simulink model "CoETM_ClgDem"  (R2016b)
settings: configuration reference "CodeGenConfigSet" (kept outside this file)
values from neighbouring files (symbols this model uses):
  CoETM_AfterRun2_C = Calibration.Parameter    [init_CoETM_ClgDem.m]
  CoETM_facAftRun2_C = Calibration.Parameter    [init_CoETM_ClgDem.m]
  CoETM_facClgAftRun_CUR = Calibration.Parameter    [init_CoETM_ClgDem.m]
  CoETM_facClgAftRun_CURX = Calibration.Parameter    [init_CoETM_ClgDem.m]
  CoETM_facClgDem_DT_C = Calibration.Parameter    [init_CoETM_ClgDem.m]
  CoETM_rClgAftRun_MAP = Calibration.Parameter    [init_CoETM_ClgDem.m]
  CoETM_rClgAftRun_MAPX = Calibration.Parameter    [init_CoETM_ClgDem.m]
  CoETM_rClgAftRun_MAPY = Calibration.Parameter    [init_CoETM_ClgDem.m]
  CoETM_rClgDemFan_CUR = Calibration.Parameter    [init_CoETM_ClgDem.m]
  CoETM_rClgDemFan_CURX = Calibration.Parameter    [init_CoETM_ClgDem.m]
  CoETM_rClgDemMax_C = Calibration.Parameter    [init_CoETM_ClgDem.m]
  CoETM_rClgDemMin_C = Calibration.Parameter    [init_CoETM_ClgDem.m]
  CoETM_rClgDemT_CUR = Calibration.Parameter    [init_CoETM_ClgDem.m]
  CoETM_rClgDemT_CURX = Calibration.Parameter    [init_CoETM_ClgDem.m]
  CoETM_rClgKi_CUR = Calibration.Parameter    [init_CoETM_ClgDem.m]
  CoETM_rClgKi_CURX = Calibration.Parameter    [init_CoETM_ClgDem.m]
  CoETM_rClgKp_CUR = Calibration.Parameter    [init_CoETM_ClgDem.m]
  CoETM_rClgKp_CURX = Calibration.Parameter    [init_CoETM_ClgDem.m]
  CoETM_RmpSlpNeg_C = Calibration.Parameter    [init_CoETM_ClgDem.m]
  CoETM_RmpSlpPos_C = Calibration.Parameter    [init_CoETM_ClgDem.m]
  CoETM_swtCTTCTL_SY_C = Calibration.Parameter    [init_CoETM_ClgDem.m]
  CoETM_swtSrc_C = Calibration.Parameter    [init_CoETM_ClgDem.m]
  CoETM_tAftRunAbrt_C = Calibration.Parameter    [init_CoETM_ClgDem.m]
  CoETM_tClntStg1Max_C = Calibration.Parameter    [init_CoETM_ClgDem.m]
  CoETM_tClntStg1Min_C = Calibration.Parameter    [init_CoETM_ClgDem.m]
  CoETM_tClntStg2Max_C = Calibration.Parameter    [init_CoETM_ClgDem.m]
  CoETM_tClntStg2Min_C = Calibration.Parameter    [init_CoETM_ClgDem.m]
  CoETM_tDvtMax_C = Calibration.Parameter    [init_CoETM_ClgDem.m]
  CoETM_tDvtMin_C = Calibration.Parameter    [init_CoETM_ClgDem.m]
  CoETM_tDvtStg0_C = Calibration.Parameter    [init_CoETM_ClgDem.m]
  CoETM_tDvtStg1_C = Calibration.Parameter    [init_CoETM_ClgDem.m]
  CoETM_tDvtStg2_C = Calibration.Parameter    [init_CoETM_ClgDem.m]
  CoETM_tEngOutSubsOff_C = Calibration.Parameter    [init_CoETM_ClgDem.m]
  CoETM_tiClgAftRun2_MAP = Calibration.Parameter    [init_CoETM_ClgDem.m]
  CoETM_tiClgAftRun2_MAPX = Calibration.Parameter    [init_CoETM_ClgDem.m]
  CoETM_tiClgAftRun2_MAPY = Calibration.Parameter    [init_CoETM_ClgDem.m]
  CoETM_tiClgAftRun_MAP = Calibration.Parameter    [init_CoETM_ClgDem.m]
  CoETM_tiClgAftRun_MAPX = Calibration.Parameter    [init_CoETM_ClgDem.m]
  CoETM_tiClgAftRun_MAPY = Calibration.Parameter    [init_CoETM_ClgDem.m]
  CoETM_tiClgAftRunCons_MAP = Calibration.Parameter    [init_CoETM_ClgDem.m]
  CoETM_tiClgAftRunCons_MAPX = Calibration.Parameter    [init_CoETM_ClgDem.m]
  CoETM_tiClgAftRunCons_MAPY = Calibration.Parameter    [init_CoETM_ClgDem.m]
  CoETM_tiClgAftRunOil_MAP = Calibration.Parameter    [init_CoETM_ClgDem.m]
  CoETM_tiClgAftRunOil_MAPX = Calibration.Parameter    [init_CoETM_ClgDem.m]
  CoETM_tiClgAftRunTEnv_CUR = Calibration.Parameter    [init_CoETM_ClgDem.m]
  CoETM_tiClgAftRunTEnv_CURX = Calibration.Parameter    [init_CoETM_ClgDem.m]
  PRC_ZERO = fi(0,Prc_100_rate)    [init_CoETM_ClgDem.m]
undefined symbols (not defined in the file or in its folder): CoETM_ClgDem_DT, EngState_conv, FanCtl_facCorSpd_MAPX
libraries: CXLib x7
settings Model: Creator=xinchangran  LastModifiedBy=xinchangran
settings ConfigSetRef: SourceLocation=Base Workspace

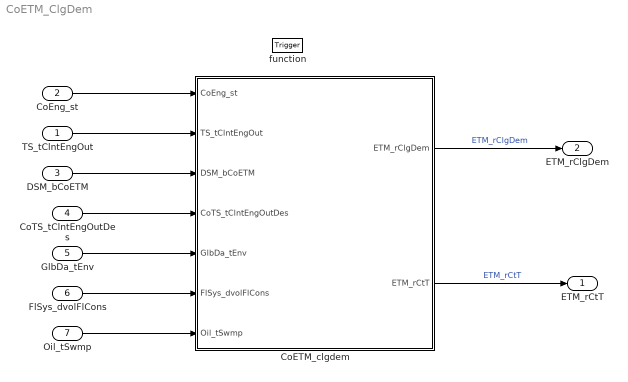
== system CoETM_ClgDem ==
  TS_tClntEngOut : Inport  Tag=deg  Description=desired coolant temperature  OutMin=-3549  OutMax=3003  OutDataTypeStr=Temp_deg
  CoEng_st : Inport  Description=Engine coordinator state  Port=2  OutDataTypeStr=Enum: EngState_conv
  DSM_bCoETM : Inport  Description=in case of coolant temperature signal error  Port=3  OutMin=0  OutMax=1  OutDataTypeStr=boolean
  CoTS_tClntEngOutDes : Inport  Tag=deg  Description=Coolant temperature of combustion engine  Port=4  OutMin=-3549  OutMax=3003  OutDataTypeStr=Temp_deg
  GlbDa_tEnv : Inport  Tag=deg  Description=environment temperature  Port=5  OutMin=-50  OutMax=150  OutDataTypeStr=Temp_deg
  FlSys_dvolFlCons : Inport  Tag=L/h  Description=Fuel consumption [l/h]  Port=6  OutMin=0  OutMax=327  OutDataTypeStr=FlCon_L_h
  Oil_tSwmp : Inport  Tag=deg  Description=Oil temperature in oil sump  Port=7  OutMin=-50  OutMax=200  OutDataTypeStr=Temp_deg
  function : TriggerPort  TriggerType=function-call  VariantControl=Variant
  CoETM_clgdem : Subsystem
  ETM_rCtT : Outport  Tag=%  Description=Energisation of electrical thermostat  OutMin=-300  OutMax=300  OutDataTypeStr=Prc_100_rate
  ETM_rClgDem : Outport  Tag=%  Description=Relative fan cooling power required by engine cooling  Port=2  OutMin=-300  OutMax=300  OutDataTypeStr=Prc_100_rate
  wires:
  CoEng_st/1 -> CoETM_clgdem/1(CoEng_st)
  TS_tClntEngOut/1 -> CoETM_clgdem/2(TS_tClntEngOut)
  DSM_bCoETM/1 -> CoETM_clgdem/3(DSM_bCoETM)
  CoTS_tClntEngOutDes/1 -> CoETM_clgdem/4(CoTS_tClntEngOutDes)
  GlbDa_tEnv/1 -> CoETM_clgdem/5(GlbDa_tEnv)
  FlSys_dvolFlCons/1 -> CoETM_clgdem/6(FlSys_dvolFlCons)
  Oil_tSwmp/1 -> CoETM_clgdem/7(Oil_tSwmp)
  CoETM_clgdem/1(ETM_rClgDem) -> ETM_rClgDem/1  "ETM_rClgDem"
  CoETM_clgdem/2(ETM_rCtT) -> ETM_rCtT/1  "ETM_rCtT"

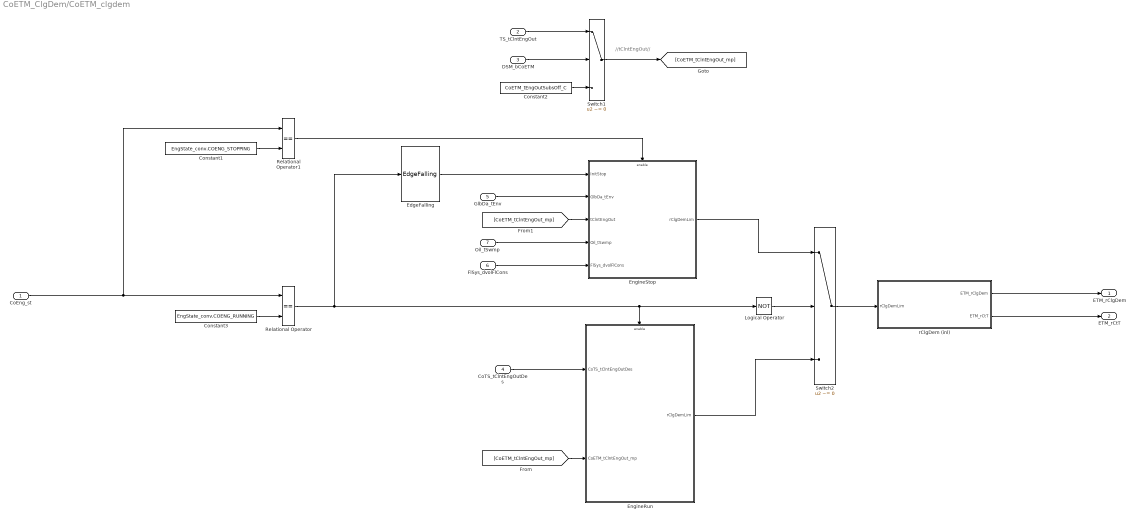
== system CoETM_ClgDem/CoETM_clgdem ==
  note: //tClntEngOut//
  CoEng_st : Inport  Description=Engine coordinator state  OutDataTypeStr=Enum: EngState_conv
  TS_tClntEngOut : Inport  Tag=deg  Description=desired coolant temperature  Port=2  OutMin=-3549  OutMax=3003  OutDataTypeStr=Temp_deg
  DSM_bCoETM : Inport  Description=in case of coolant temperature signal error  Port=3  OutMin=0  OutMax=1  OutDataTypeStr=boolean
  CoTS_tClntEngOutDes : Inport  Port=4
  GlbDa_tEnv : Inport  Port=5
  FlSys_dvolFlCons : Inport  Port=6
  Oil_tSwmp : Inport  Port=7
  Constant1 : Constant  Value=EngState_conv.COENG_STOPPING
  Constant2 : Constant  Value=CoETM_tEngOutSubsOff_C
  Constant3 : Constant  Value=EngState_conv.COENG_RUNNING
  EdgeFalling : CXLib/EdgeFalling
  "EngineRun " : Subsystem  TreatAsAtomicUnit=on
  EngineStop : Subsystem  TreatAsAtomicUnit=on
  Logical Operator : Logic  Operator=NOT  AllPortsSameDT=off  OutDataTypeStr=boolean
  Relational Operator : RelationalOperator  Operator===  OutDataTypeStr=boolean  RndMeth=Simplest
  Relational Operator1 : RelationalOperator  Operator===  OutDataTypeStr=boolean  RndMeth=Simplest
  Switch1 : Switch  Criteria=u2 ~= 0  SaturateOnIntegerOverflow=on  InputSameDT=on
  Switch2 : Switch  Criteria=u2 ~= 0  SaturateOnIntegerOverflow=on  InputSameDT=on
  rClgDem (inl) : Subsystem
  ETM_rClgDem : Outport
  ETM_rCtT : Outport  Port=2
  wires:
  Logical Operator/1 -> Switch2/2
  Relational Operator1/1 -> EngineStop/Enable
  Relational Operator/1 -> EdgeFalling/1, Logical Operator/1, "EngineRun "/Enable
  Switch2/1 -> rClgDem (inl)/1(rClgDemLim)
  FlSys_dvolFlCons/1 -> EngineStop/5(FlSys_dvolFlCons)
  EngineStop/1(rClgDemLim) -> Switch2/1
  Switch1/1 -> [CoETM_tClntEngOut_mp]
  rClgDem (inl)/1(ETM_rClgDem) -> ETM_rClgDem/1
  rClgDem (inl)/2(ETM_rCtT) -> ETM_rCtT/1
  [CoETM_tClntEngOut_mp] -> "EngineRun "/2(CoETM_tClntEngOut_mp)
  Constant3/1 -> Relational Operator/2
  [CoETM_tClntEngOut_mp] -> EngineStop/3(tClntEngOut)
  EdgeFalling/1 -> EngineStop/1(InitStop)
  Constant2/1 -> Switch1/3
  GlbDa_tEnv/1 -> EngineStop/2(GlbDa_tEnv)
  CoTS_tClntEngOutDes/1 -> "EngineRun "/1(CoTS_tClntEngOutDes)
  CoEng_st/1 -> Relational Operator1/1, Relational Operator/1
  "EngineRun "/1(rClgDemLim) -> Switch2/3
  DSM_bCoETM/1 -> Switch1/2
  TS_tClntEngOut/1 -> Switch1/1
  Oil_tSwmp/1 -> EngineStop/4(Oil_tSwmp)
  Constant1/1 -> Relational Operator1/2

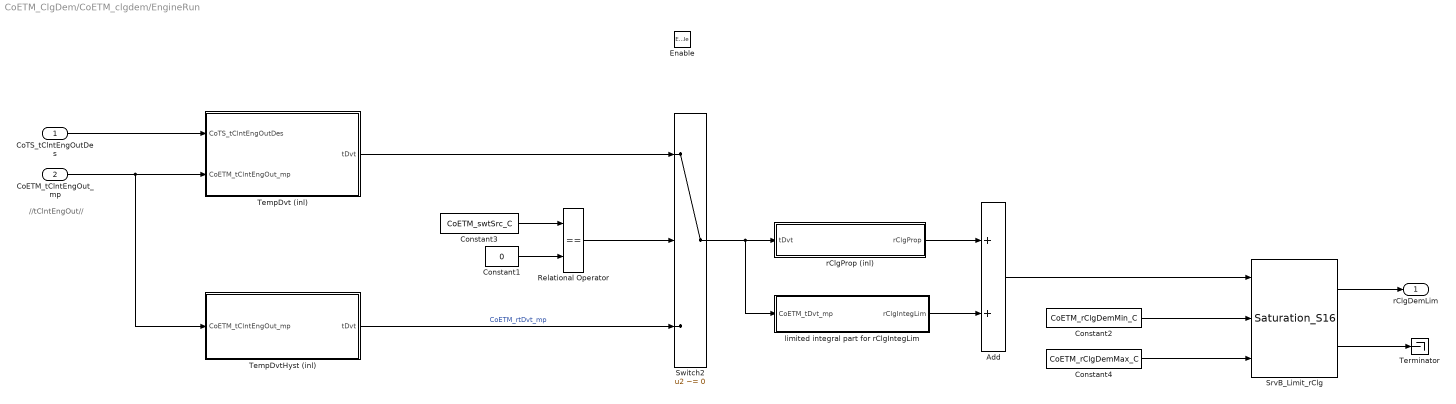
== system CoETM_ClgDem/CoETM_clgdem/EngineRun  ==
  note: //tClntEngOut//
  CoTS_tClntEngOutDes : Inport
  CoETM_tClntEngOut_mp : Inport  Port=2
  Enable : EnablePort
  Add : Sum  OutDataTypeStr=Inherit: Inherit via back propagation  SaturateOnIntegerOverflow=on
  Constant1 : Constant  Value=0
  Constant2 : Constant  Value=CoETM_rClgDemMin_C
  Constant3 : Constant  Value=CoETM_swtSrc_C
  Constant4 : Constant  Value=CoETM_rClgDemMax_C
  Relational Operator : RelationalOperator  Operator===  OutDataTypeStr=boolean  RndMeth=Simplest
  SrvB_Limit_rClg : CXLib/Saturation_S16
  Switch2 : Switch  Criteria=u2 ~= 0  SaturateOnIntegerOverflow=on  InputSameDT=on
  TempDvt (inl) : Subsystem  TreatAsAtomicUnit=on
  TempDvtHyst (inl) : Subsystem  TreatAsAtomicUnit=on
  Terminator : Terminator
  limited integral part for rClgIntegLim : Subsystem
  rClgProp (inl) : Subsystem  TreatAsAtomicUnit=on
  rClgDemLim : Outport
  wires:
  Constant3/1 -> Relational Operator/1
  Constant1/1 -> Relational Operator/2
  rClgProp (inl)/1(rClgProp) -> Add/1
  Add/1 -> SrvB_Limit_rClg/1
  SrvB_Limit_rClg/2 -> Terminator/1
  SrvB_Limit_rClg/1 -> rClgDemLim/1
  CoTS_tClntEngOutDes/1 -> TempDvt (inl)/1(CoTS_tClntEngOutDes)
  TempDvt (inl)/1(tDvt) -> Switch2/1
  TempDvtHyst (inl)/1(tDvt) -> Switch2/3  "CoETM_rtDvt_mp"
  CoETM_tClntEngOut_mp/1 -> TempDvtHyst (inl)/1(CoETM_tClntEngOut_mp), TempDvt (inl)/2(CoETM_tClntEngOut_mp)
  Relational Operator/1 -> Switch2/2
  Constant2/1 -> SrvB_Limit_rClg/2
  Constant4/1 -> SrvB_Limit_rClg/3
  limited integral part for rClgIntegLim/1(rClgIntegLim) -> Add/2
  Switch2/1 -> limited integral part for rClgIntegLim/1(CoETM_tDvt_mp), rClgProp (inl)/1(tDvt)

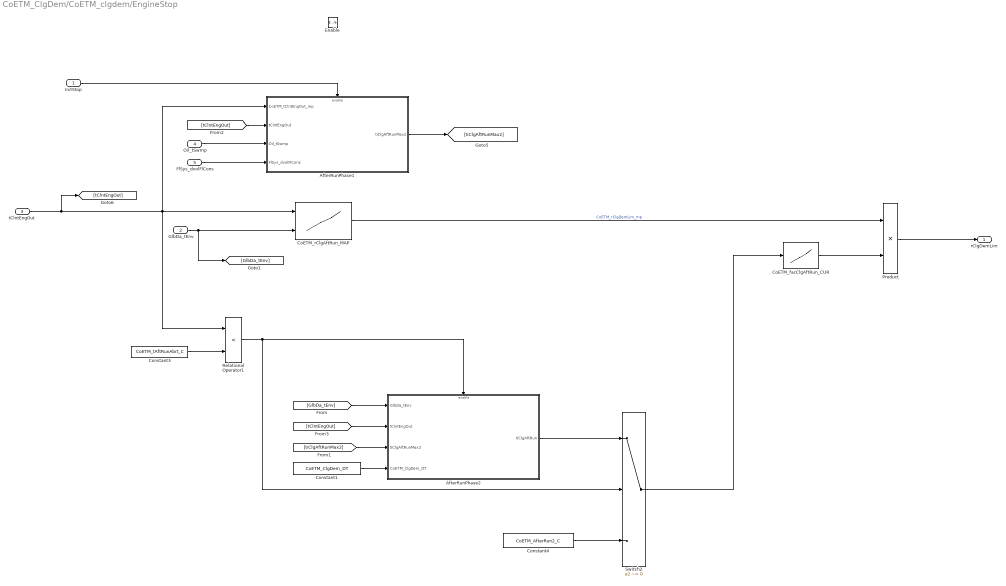
== system CoETM_ClgDem/CoETM_clgdem/EngineStop ==
  InitStop : Inport
  GlbDa_tEnv : Inport  Port=2
  tClntEngOut : Inport  Port=3
  Oil_tSwmp : Inport  Port=4
  FlSys_dvolFlCons : Inport  Port=5
  Enable : EnablePort
  AfterRunPhase1 : Subsystem  TreatAsAtomicUnit=on
  AfterRunPhase2 : Subsystem
  CoETM_facClgAftRun_CUR : Lookup_n-D  NumberOfTableDimensions=1  BreakpointsForDimension1=CoETM_facClgAftRun_CURX  BreakpointsForDimension2=FanCtl_facCorSpd_MAPX  IndexSearchMethod=Linear search  BeginIndexSearchUsingPreviousIndexResult=on  Table=CoETM_facClgAftRun_CUR  ExtrapMethod=Clip  UseLastTableValue=on  InternalRulePriority=Speed  OutDataTypeStr=Inherit: Inherit via back propagation  SaturateOnIntegerOverflow=on
  CoETM_rClgAftRun_MAP : Lookup_n-D  BreakpointsForDimension1=CoETM_rClgAftRun_MAPY  BreakpointsForDimension2=CoETM_rClgAftRun_MAPX  IndexSearchMethod=Linear search  BeginIndexSearchUsingPreviousIndexResult=on  Table=CoETM_rClgAftRun_MAP  ExtrapMethod=Clip  UseLastTableValue=on  InternalRulePriority=Speed  OutDataTypeStr=Inherit: Inherit via back propagation  SaturateOnIntegerOverflow=on
  Constant1 : Constant  Value=CoETM_ClgDem_DT  OutDataTypeStr=Inherit: Inherit via back propagation
  Constant3 : Constant  Value=CoETM_tAftRunAbrt_C
  Constant4 : Constant  Value=CoETM_AfterRun2_C
  Product : Product  OutDataTypeStr=Inherit: Inherit via back propagation  SaturateOnIntegerOverflow=on
  Relational Operator1 : RelationalOperator  Operator=<  OutDataTypeStr=boolean  RndMeth=Simplest
  Switch2 : Switch  Criteria=u2 ~= 0  SaturateOnIntegerOverflow=on  InputSameDT=on
  rClgDemLim : Outport
  wires:
  tClntEngOut/1 -> [tClntEngOut], Relational Operator1/1, AfterRunPhase1/1(CoETM_tClntEngOut_mp), CoETM_rClgAftRun_MAP/1
  GlbDa_tEnv/1 -> [GlbDa_tEnv], CoETM_rClgAftRun_MAP/2
  CoETM_rClgAftRun_MAP/1 -> Product/1  "CoETM_rClgDemLim_mp"
  CoETM_facClgAftRun_CUR/1 -> Product/2
  Product/1 -> rClgDemLim/1
  InitStop/1 -> AfterRunPhase1/Enable
  Constant3/1 -> Relational Operator1/2
  AfterRunPhase1/1(tiClgAftRunMax2) -> [tiClgAftRunMax2]
  FlSys_dvolFlCons/1 -> AfterRunPhase1/4(FlSys_dvolFlCons)
  Oil_tSwmp/1 -> AfterRunPhase1/3(Oil_tSwmp)
  [tClntEngOut] -> AfterRunPhase1/2(tClntEngOut)
  [GlbDa_tEnv] -> AfterRunPhase2/1(GlbDa_tEnv)
  [tiClgAftRunMax2] -> AfterRunPhase2/3(tiClgAftRunMax2)
  [tClntEngOut] -> AfterRunPhase2/2(tClntEngOut)
  Constant1/1 -> AfterRunPhase2/4(CoETM_ClgDem_DT)
  Constant4/1 -> Switch2/3
  AfterRunPhase2/1(tiClgAftRun) -> Switch2/1
  Relational Operator1/1 -> Switch2/2, AfterRunPhase2/Enable
  Switch2/1 -> CoETM_facClgAftRun_CUR/1

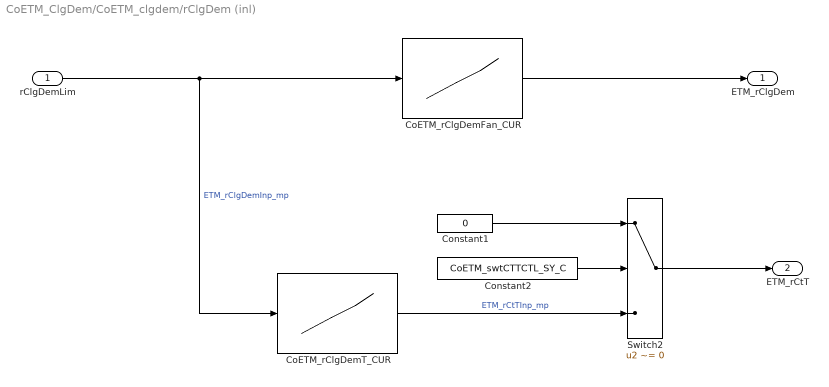
== system CoETM_ClgDem/CoETM_clgdem/rClgDem (inl) ==
  rClgDemLim : Inport
  CoETM_rClgDemFan_CUR : Lookup_n-D  NumberOfTableDimensions=1  BreakpointsForDimension1=CoETM_rClgDemFan_CURX  BreakpointsForDimension2=FanCtl_facCorSpd_MAPX  IndexSearchMethod=Linear search  BeginIndexSearchUsingPreviousIndexResult=on  Table=CoETM_rClgDemFan_CUR  ExtrapMethod=Clip  UseLastTableValue=on  InternalRulePriority=Speed  OutDataTypeStr=Inherit: Inherit via back propagation  SaturateOnIntegerOverflow=on
  CoETM_rClgDemT_CUR : Lookup_n-D  NumberOfTableDimensions=1  BreakpointsForDimension1=CoETM_rClgDemT_CURX  BreakpointsForDimension2=FanCtl_facCorSpd_MAPX  IndexSearchMethod=Linear search  BeginIndexSearchUsingPreviousIndexResult=on  Table=CoETM_rClgDemT_CUR  ExtrapMethod=Clip  UseLastTableValue=on  InternalRulePriority=Speed  OutDataTypeStr=Inherit: Inherit via back propagation  SaturateOnIntegerOverflow=on
  Constant1 : Constant  Value=0  OutDataTypeStr=Inherit: Inherit via back propagation
  Constant2 : Constant  Value=CoETM_swtCTTCTL_SY_C
  Switch2 : Switch  Criteria=u2 ~= 0  SaturateOnIntegerOverflow=on  InputSameDT=on
  ETM_rClgDem : Outport
  ETM_rCtT : Outport  Port=2
  wires:
  CoETM_rClgDemFan_CUR/1 -> ETM_rClgDem/1
  rClgDemLim/1 -> CoETM_rClgDemT_CUR/1, CoETM_rClgDemFan_CUR/1  "ETM_rClgDemInp_mp"
  CoETM_rClgDemT_CUR/1 -> Switch2/3  "ETM_rCtTInp_mp"
  Switch2/1 -> ETM_rCtT/1
  Constant2/1 -> Switch2/2
  Constant1/1 -> Switch2/1

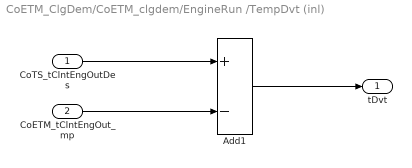
== system CoETM_ClgDem/CoETM_clgdem/EngineRun /TempDvt (inl) ==
  CoTS_tClntEngOutDes : Inport
  CoETM_tClntEngOut_mp : Inport  Port=2
  Add1 : Sum  Inputs=+-  OutDataTypeStr=Inherit: Inherit via back propagation  SaturateOnIntegerOverflow=on
  tDvt : Outport
  wires:
  CoTS_tClntEngOutDes/1 -> Add1/1
  CoETM_tClntEngOut_mp/1 -> Add1/2
  Add1/1 -> tDvt/1

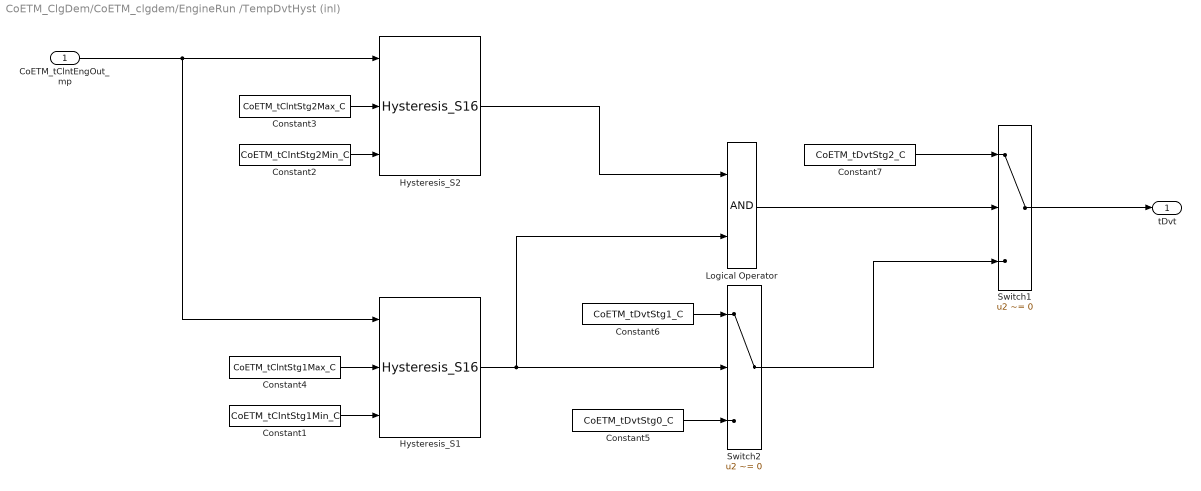
== system CoETM_ClgDem/CoETM_clgdem/EngineRun /TempDvtHyst (inl) ==
  CoETM_tClntEngOut_mp : Inport
  Constant1 : Constant  Value=CoETM_tClntStg1Min_C
  Constant2 : Constant  Value=CoETM_tClntStg2Min_C
  Constant3 : Constant  Value=CoETM_tClntStg2Max_C
  Constant4 : Constant  Value=CoETM_tClntStg1Max_C
  Constant5 : Constant  Value=CoETM_tDvtStg0_C
  Constant6 : Constant  Value=CoETM_tDvtStg1_C
  Constant7 : Constant  Value=CoETM_tDvtStg2_C
  Hysteresis_S1 : CXLib/Hysteresis_S16
  Hysteresis_S2 : CXLib/Hysteresis_S16
  Logical Operator : Logic  AllPortsSameDT=off  OutDataTypeStr=boolean
  Switch1 : Switch  Criteria=u2 ~= 0  SaturateOnIntegerOverflow=on  InputSameDT=on
  Switch2 : Switch  Criteria=u2 ~= 0  SaturateOnIntegerOverflow=on  InputSameDT=on
  tDvt : Outport
  wires:
  Constant4/1 -> Hysteresis_S1/2
  Constant1/1 -> Hysteresis_S1/3
  Constant3/1 -> Hysteresis_S2/2
  Constant2/1 -> Hysteresis_S2/3
  Constant5/1 -> Switch2/3
  Constant6/1 -> Switch2/1
  Switch2/1 -> Switch1/3
  Constant7/1 -> Switch1/1
  Logical Operator/1 -> Switch1/2
  Hysteresis_S1/1 -> Logical Operator/2, Switch2/2
  Hysteresis_S2/1 -> Logical Operator/1
  CoETM_tClntEngOut_mp/1 -> Hysteresis_S1/1, Hysteresis_S2/1
  Switch1/1 -> tDvt/1

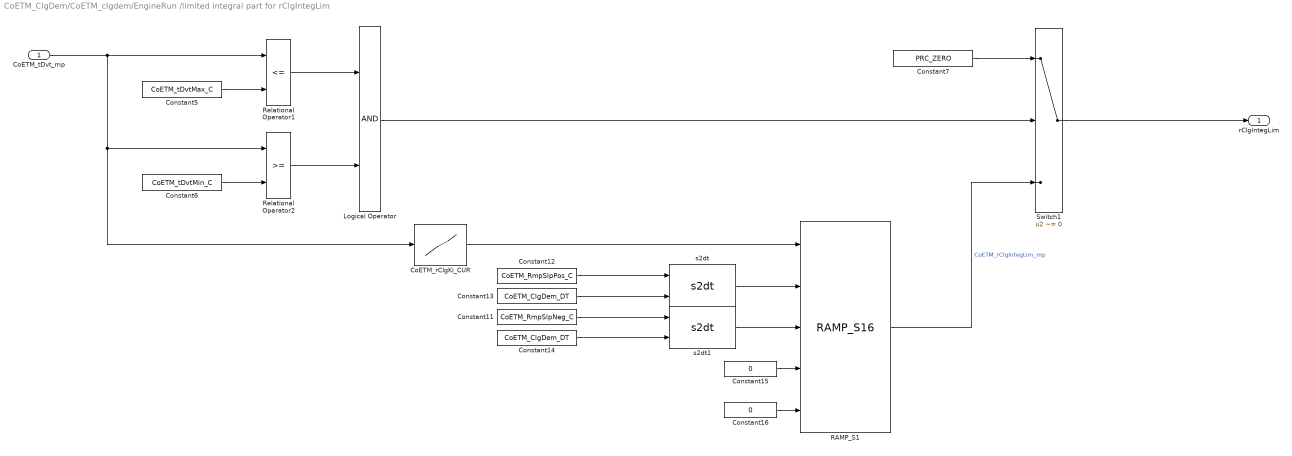
== system CoETM_ClgDem/CoETM_clgdem/EngineRun /limited integral part for rClgIntegLim ==
  CoETM_tDvt_mp : Inport
  CoETM_rClgKi_CUR : Lookup_n-D  NumberOfTableDimensions=1  BreakpointsForDimension1=CoETM_rClgKi_CURX  BreakpointsForDimension2=FanCtl_facCorSpd_MAPX  IndexSearchMethod=Linear search  BeginIndexSearchUsingPreviousIndexResult=on  Table=CoETM_rClgKi_CUR  ExtrapMethod=Clip  UseLastTableValue=on  InternalRulePriority=Speed  OutDataTypeStr=Inherit: Inherit via back propagation  SaturateOnIntegerOverflow=on
  Constant11 : Constant  Value=CoETM_RmpSlpNeg_C
  Constant12 : Constant  Value=CoETM_RmpSlpPos_C
  Constant13 : Constant  Value=CoETM_ClgDem_DT
  Constant14 : Constant  Value=CoETM_ClgDem_DT
  Constant15 : Constant  Value=0  OutDataTypeStr=Inherit: Inherit via back propagation
  Constant16 : Constant  Value=0  OutDataTypeStr=Inherit: Inherit via back propagation
  Constant5 : Constant  Value=CoETM_tDvtMax_C
  Constant6 : Constant  Value=CoETM_tDvtMin_C
  Constant7 : Constant  Value=PRC_ZERO  OutDataTypeStr=Inherit: Inherit via back propagation
  Logical Operator : Logic  AllPortsSameDT=off  OutDataTypeStr=boolean
  RAMP_S1 : CXLib/RAMP_S16
  Relational Operator1 : RelationalOperator  Operator=<=  OutDataTypeStr=boolean  RndMeth=Simplest
  Relational Operator2 : RelationalOperator  OutDataTypeStr=boolean  RndMeth=Simplest
  Switch1 : Switch  Criteria=u2 ~= 0  SaturateOnIntegerOverflow=on  InputSameDT=on
  s2dt : CXLib/s2dt
  s2dt1 : CXLib/s2dt
  rClgIntegLim : Outport
  wires:
  Constant7/1 -> Switch1/1
  Logical Operator/1 -> Switch1/2
  Constant6/1 -> Relational Operator2/2
  Relational Operator2/1 -> Logical Operator/2
  CoETM_tDvt_mp/1 -> CoETM_rClgKi_CUR/1, Relational Operator2/1, Relational Operator1/1
  RAMP_S1/1 -> Switch1/3  "CoETM_rClgIntegLim_mp"
  Constant5/1 -> Relational Operator1/2
  Relational Operator1/1 -> Logical Operator/1
  s2dt/1 -> RAMP_S1/2
  Constant11/1 -> s2dt1/1
  Constant13/1 -> s2dt/2
  Constant12/1 -> s2dt/1
  s2dt1/1 -> RAMP_S1/3
  CoETM_rClgKi_CUR/1 -> RAMP_S1/1
  Constant15/1 -> RAMP_S1/4
  Constant14/1 -> s2dt1/2
  Constant16/1 -> RAMP_S1/5
  Switch1/1 -> rClgIntegLim/1

== system CoETM_ClgDem/CoETM_clgdem/EngineRun /rClgProp (inl) ==
  tDvt : Inport
  CoETM_rClgKp_CUR : Lookup_n-D  NumberOfTableDimensions=1  BreakpointsForDimension1=CoETM_rClgKp_CURX  BreakpointsForDimension2=FanCtl_facCorSpd_MAPX  IndexSearchMethod=Linear search  BeginIndexSearchUsingPreviousIndexResult=on  Table=CoETM_rClgKp_CUR  ExtrapMethod=Clip  UseLastTableValue=on  InternalRulePriority=Speed  OutDataTypeStr=Inherit: Inherit via back propagation  SaturateOnIntegerOverflow=on
  rClgProp : Outport
  wires:
  tDvt/1 -> CoETM_rClgKp_CUR/1
  CoETM_rClgKp_CUR/1 -> rClgProp/1

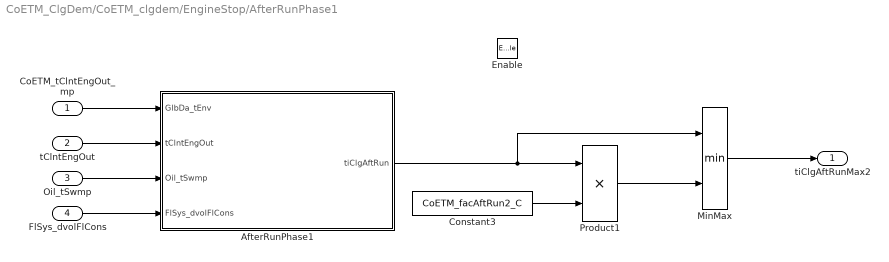
== system CoETM_ClgDem/CoETM_clgdem/EngineStop/AfterRunPhase1 ==
  CoETM_tClntEngOut_mp : Inport
  tClntEngOut : Inport  Port=2
  Oil_tSwmp : Inport  Port=3
  FlSys_dvolFlCons : Inport  Port=4
  Enable : EnablePort
  AfterRunPhase1 : Subsystem
  Constant3 : Constant  Value=CoETM_facAftRun2_C
  MinMax : MinMax  Inputs=2
  Product1 : Product  OutDataTypeStr=Inherit: Inherit via back propagation  SaturateOnIntegerOverflow=on
  tiClgAftRunMax2 : Outport
  wires:
  AfterRunPhase1/1("tiClgAftRun ") -> MinMax/1, Product1/1
  Constant3/1 -> Product1/2
  Product1/1 -> MinMax/2
  MinMax/1 -> tiClgAftRunMax2/1
  CoETM_tClntEngOut_mp/1 -> AfterRunPhase1/1(GlbDa_tEnv)
  tClntEngOut/1 -> AfterRunPhase1/2(tClntEngOut)
  Oil_tSwmp/1 -> AfterRunPhase1/3(Oil_tSwmp)
  FlSys_dvolFlCons/1 -> AfterRunPhase1/4(FlSys_dvolFlCons)

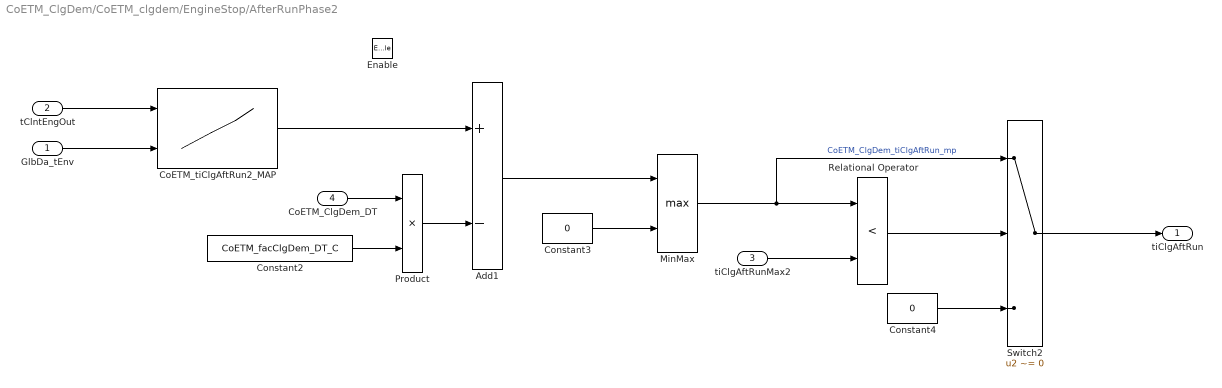
== system CoETM_ClgDem/CoETM_clgdem/EngineStop/AfterRunPhase2 ==
  GlbDa_tEnv : Inport
  tClntEngOut : Inport  Port=2
  tiClgAftRunMax2 : Inport  Port=3
  CoETM_ClgDem_DT : Inport  Port=4
  Enable : EnablePort
  Add1 : Sum  Inputs=+-  OutDataTypeStr=Inherit: Inherit via back propagation  SaturateOnIntegerOverflow=on
  CoETM_tiClgAftRun2_MAP : Lookup_n-D  BreakpointsForDimension1=CoETM_tiClgAftRun2_MAPY  BreakpointsForDimension2=CoETM_tiClgAftRun2_MAPX  IndexSearchMethod=Linear search  BeginIndexSearchUsingPreviousIndexResult=on  Table=CoETM_tiClgAftRun2_MAP  ExtrapMethod=Clip  UseLastTableValue=on  InternalRulePriority=Speed  OutDataTypeStr=Inherit: Inherit via back propagation  SaturateOnIntegerOverflow=on
  Constant2 : Constant  Value=CoETM_facClgDem_DT_C
  Constant3 : Constant  Value=0  OutDataTypeStr=Inherit: Inherit via back propagation
  Constant4 : Constant  Value=0  OutDataTypeStr=Inherit: Inherit via back propagation
  MinMax : MinMax  Function=max  Inputs=2  OutDataTypeStr=Inherit: Inherit via back propagation  SaturateOnIntegerOverflow=on
  Product : Product  OutDataTypeStr=Inherit: Inherit via back propagation  SaturateOnIntegerOverflow=on
  Relational Operator : RelationalOperator  Operator=<  OutDataTypeStr=boolean  RndMeth=Simplest
  Switch2 : Switch  Criteria=u2 ~= 0  SaturateOnIntegerOverflow=on  InputSameDT=on
  tiClgAftRun : Outport
  wires:
  Constant3/1 -> MinMax/2
  tClntEngOut/1 -> CoETM_tiClgAftRun2_MAP/1
  GlbDa_tEnv/1 -> CoETM_tiClgAftRun2_MAP/2
  MinMax/1 -> Switch2/1, Relational Operator/1  "CoETM_ClgDem_tiClgAftRun_mp"
  CoETM_tiClgAftRun2_MAP/1 -> Add1/1
  Product/1 -> Add1/2
  CoETM_ClgDem_DT/1 -> Product/1
  Constant2/1 -> Product/2
  Add1/1 -> MinMax/1
  tiClgAftRunMax2/1 -> Relational Operator/2
  Relational Operator/1 -> Switch2/2
  Constant4/1 -> Switch2/3
  Switch2/1 -> tiClgAftRun/1

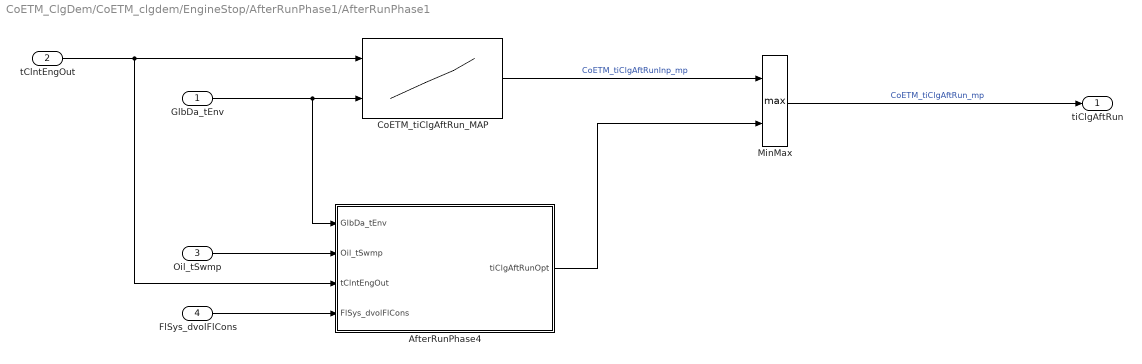
== system CoETM_ClgDem/CoETM_clgdem/EngineStop/AfterRunPhase1/AfterRunPhase1 ==
  GlbDa_tEnv : Inport
  tClntEngOut : Inport  Port=2
  Oil_tSwmp : Inport  Port=3
  FlSys_dvolFlCons : Inport  Port=4
  AfterRunPhase4 : Subsystem  TreatAsAtomicUnit=on
  CoETM_tiClgAftRun_MAP : Lookup_n-D  BreakpointsForDimension1=CoETM_tiClgAftRun_MAPY  BreakpointsForDimension2=CoETM_tiClgAftRun_MAPX  IndexSearchMethod=Linear search  BeginIndexSearchUsingPreviousIndexResult=on  Table=CoETM_tiClgAftRun_MAP  ExtrapMethod=Clip  UseLastTableValue=on  InternalRulePriority=Speed  OutDataTypeStr=Inherit: Inherit via back propagation  SaturateOnIntegerOverflow=on
  MinMax : MinMax  Function=max  Inputs=2  OutDataTypeStr=Inherit: Inherit via back propagation  SaturateOnIntegerOverflow=on
  "tiClgAftRun " : Outport
  wires:
  AfterRunPhase4/1("tiClgAftRunOpt ") -> MinMax/2
  MinMax/1 -> "tiClgAftRun "/1  "CoETM_tiClgAftRun_mp"
  GlbDa_tEnv/1 -> AfterRunPhase4/1(GlbDa_tEnv), CoETM_tiClgAftRun_MAP/2
  tClntEngOut/1 -> AfterRunPhase4/3(tClntEngOut), CoETM_tiClgAftRun_MAP/1
  CoETM_tiClgAftRun_MAP/1 -> MinMax/1  "CoETM_tiClgAftRunInp_mp"
  Oil_tSwmp/1 -> AfterRunPhase4/2(Oil_tSwmp)
  FlSys_dvolFlCons/1 -> AfterRunPhase4/4(FlSys_dvolFlCons)

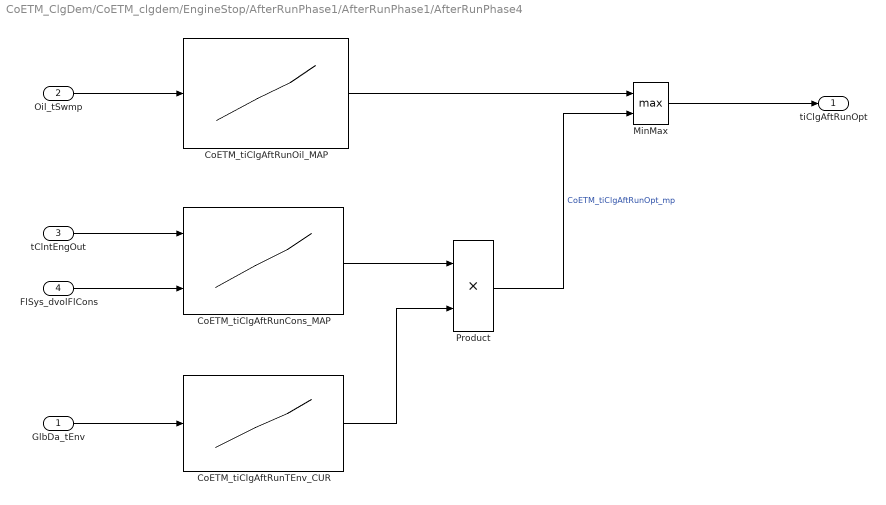
== system CoETM_ClgDem/CoETM_clgdem/EngineStop/AfterRunPhase1/AfterRunPhase1/AfterRunPhase4 ==
  GlbDa_tEnv : Inport
  Oil_tSwmp : Inport  Port=2
  tClntEngOut : Inport  Port=3
  FlSys_dvolFlCons : Inport  Port=4
  CoETM_tiClgAftRunCons_MAP : Lookup_n-D  BreakpointsForDimension1=CoETM_tiClgAftRunCons_MAPY  BreakpointsForDimension2=CoETM_tiClgAftRunCons_MAPX  IndexSearchMethod=Linear search  BeginIndexSearchUsingPreviousIndexResult=on  Table=CoETM_tiClgAftRunCons_MAP  ExtrapMethod=Clip  UseLastTableValue=on  InternalRulePriority=Speed  OutDataTypeStr=Inherit: Inherit via back propagation  SaturateOnIntegerOverflow=on
  CoETM_tiClgAftRunOil_MAP : Lookup_n-D  NumberOfTableDimensions=1  BreakpointsForDimension1=CoETM_tiClgAftRunOil_MAPX  BreakpointsForDimension2=FanCtl_facCorSpd_MAPX  IndexSearchMethod=Linear search  BeginIndexSearchUsingPreviousIndexResult=on  Table=CoETM_tiClgAftRunOil_MAP  ExtrapMethod=Clip  UseLastTableValue=on  InternalRulePriority=Speed  OutDataTypeStr=Inherit: Inherit via back propagation  SaturateOnIntegerOverflow=on
  CoETM_tiClgAftRunTEnv_CUR : Lookup_n-D  NumberOfTableDimensions=1  BreakpointsForDimension1=CoETM_tiClgAftRunTEnv_CURX  BreakpointsForDimension2=FanCtl_facCorSpd_MAPX  IndexSearchMethod=Linear search  BeginIndexSearchUsingPreviousIndexResult=on  Table=CoETM_tiClgAftRunTEnv_CUR  ExtrapMethod=Clip  UseLastTableValue=on  InternalRulePriority=Speed  OutDataTypeStr=Inherit: Inherit via back propagation  SaturateOnIntegerOverflow=on
  MinMax : MinMax  Function=max  Inputs=2
  Product : Product  OutDataTypeStr=Inherit: Inherit via back propagation  SaturateOnIntegerOverflow=on
  "tiClgAftRunOpt " : Outport
  wires:
  FlSys_dvolFlCons/1 -> CoETM_tiClgAftRunCons_MAP/2
  MinMax/1 -> "tiClgAftRunOpt "/1
  Oil_tSwmp/1 -> CoETM_tiClgAftRunOil_MAP/1
  CoETM_tiClgAftRunOil_MAP/1 -> MinMax/1
  CoETM_tiClgAftRunCons_MAP/1 -> Product/1
  GlbDa_tEnv/1 -> CoETM_tiClgAftRunTEnv_CUR/1
  tClntEngOut/1 -> CoETM_tiClgAftRunCons_MAP/1
  CoETM_tiClgAftRunTEnv_CUR/1 -> Product/2
  Product/1 -> MinMax/2  "CoETM_tiClgAftRunOpt_mp"
